simulink model "bio_matfunc_misalign_transform"  (R2017b)
settings: Solver=VariableStepAuto  StartTime=0.0  StopTime=10.0  RelTol=1e-3
settings Model: Creator=ktrinh  LastModifiedBy=ktrinh

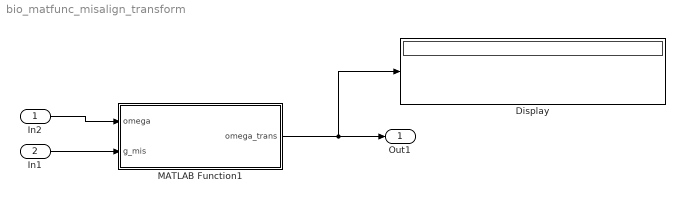
== system bio_matfunc_misalign_transform ==
  In2 : Inport  OutDataTypeStr=double  PortDimensions=1
  In1 : Inport  Port=2  OutDataTypeStr=double  PortDimensions=3
  Display : Display
  MATLAB Function1 : MATLAB Function  TreatAsAtomicUnit=on
  Out1 : Outport
  wires:
  In2/1 -> MATLAB Function1/1(omega)
  MATLAB Function1/1(omega_trans) -> Display/1, Out1/1
  In1/1 -> MATLAB Function1/2(g_mis)

== matlab function bio_matfunc_misalign_transform/MATLAB Function1 ==
  data: omega input; omega_trans output; g_mis input
function omega_trans = misalign_transform(omega,g_mis)
%#codegen

x = g_mis(1);
y = g_mis(2);
z = g_mis(3);

R = eye(3) - [0 -z y; z 0 -x; -y x 0];

omega_trans = R*omega;
